simulink model "test1"  (R2014a)
settings: Solver=ode4  StartTime=0.0  StopTime=20  FixedStep=0.1  RelTol=1e-3
settings Model: Creator=ses  LastModifiedBy=ses
settings RTWCC: GenCodeOnly=on  GenerateReport=on  Toolchain=Microsoft Windows SDK v7.1 | nmake (64-bit Windows)  LaunchReport=on

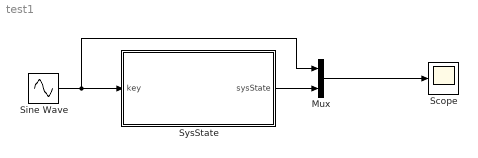
== system test1 ==
  Mux : Mux  Inputs=2
  Scope : Scope
  Sine Wave : Sin  SampleTime=0
  SysState : Stateflow chart  TreatAsAtomicUnit=on
  wires:
  Sine Wave/1 -> Mux/1, SysState/1(key)
  SysState/1(sysState) -> Mux/2
  Mux/1 -> Scope/1

== stateflow chart test1/SysState ==
  state Idle
    % Idle mode
    entry:
    sysState = 0;
  state Run
    % Running
    entry:
    sysState = 1;
  (default) -> Idle
  (junction 13) -> Idle
  Idle -> Run : % Key on
      | [key > 0]
  Run -> (junction 5)
  (junction 11) -> (junction 13)
  (junction 5) -> (junction 9)
  (junction 9) -> (junction 11) : % Key off
      | [key <= 0]
  data: key input; sysState output
